simulink model "PIDcontrol_sim"  (R2017a)
settings: Solver=FixedStepAuto  StartTime=0.0  StopTime=Endtime  FixedStep=0.1  RelTol=1e-3
values from neighbouring files (symbols this model uses):
  T_f = 1/omega_c    (= 0.318309886184)    [PIDcontrol.m]
  Ts = 1    [PIDcontrol.m]
undefined symbols (not defined in the file or in its folder): Humusoft, MF644
libraries: sldrtlib x5
settings Model: Creator=CSE2017  LastModifiedBy=CSE2017

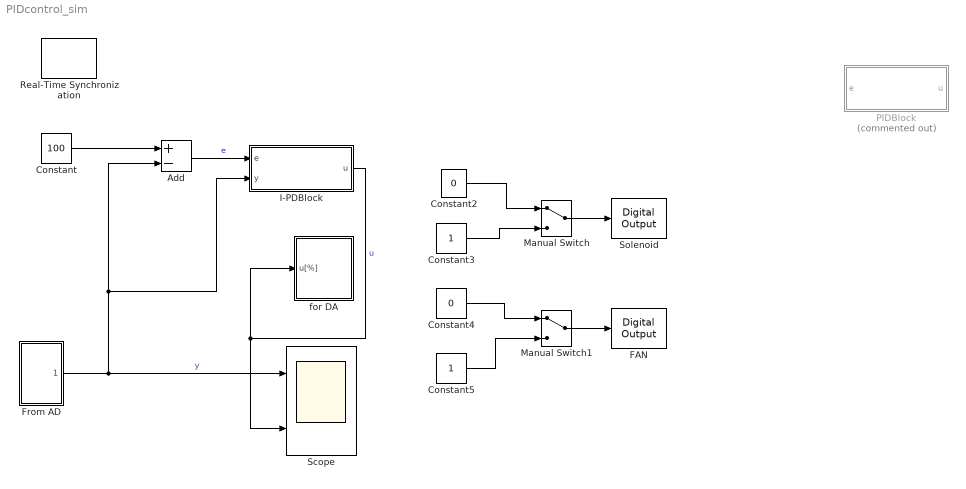
== system PIDcontrol_sim ==
  Add : Sum  Inputs=+-
  Constant : Constant  Value=100
  Constant2 : Constant  Value=0
  Constant3 : Constant
  Constant4 : Constant  Value=0
  Constant5 : Constant
  FAN : sldrtlib/Digital Output  SampleTime=Ts  MaxMissedTicks=10  ShowMissedTicks=off  YieldWhenWaiting=off  DrvName=Humusoft/MF644  DrvAddress=4294967295  DrvOptions=0  Channels=2  BitMode=1  InitialValue=0  FinalValue=1
      settings: AttributesFormatString=Humusoft\nMF644 [auto]  SourceProductName=Simulink Desktop Real-Time  SourceProductBaseCode=WT
  From AD : Subsystem
  I-PDBlock : Subsystem
  Manual Switch : ManualSwitch
  Manual Switch1 : ManualSwitch
  PIDBlock : Subsystem  Commented=on
  Real-Time Synchronization : sldrtlib/Real-Time Synchronization  SampleTime=Ts  MaxMissedTicks=10  ShowMissedTicks=off  YieldWhenWaiting=off
  Scope : Scope  NumInputPorts=2
  Solenoid : sldrtlib/Digital Output  SampleTime=Ts  MaxMissedTicks=10  ShowMissedTicks=off  YieldWhenWaiting=off  DrvName=Humusoft/MF644  DrvAddress=4294967295  DrvOptions=0  Channels=1  BitMode=1  InitialValue=0  FinalValue=0
      settings: AttributesFormatString=Humusoft\nMF644 [auto]  SourceProductName=Simulink Desktop Real-Time  SourceProductBaseCode=WT
  for DA : Subsystem
  wires:
  I-PDBlock/1(u) -> for DA/1(u[%]), Scope/2  "u"
  Constant2/1 -> Manual Switch/1
  Constant3/1 -> Manual Switch/2
  Constant4/1 -> Manual Switch1/1
  Constant5/1 -> Manual Switch1/2
  Manual Switch1/1 -> FAN/1
  Manual Switch/1 -> Solenoid/1
  From AD/1(y[deg.]) -> Add/2, I-PDBlock/2("y "), Scope/1  "y"
  Constant/1 -> Add/1
  Add/1 -> I-PDBlock/1(e)  "e"

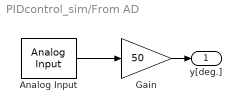
== system PIDcontrol_sim/From AD ==
  Analog Input : sldrtlib/Analog Input  SampleTime=Ts  MaxMissedTicks=10  ShowMissedTicks=off  YieldWhenWaiting=off  DrvName=Humusoft/MF644  DrvAddress=4294967295  DrvOptions=0  Channels=1  RangeMode=1  VoltRange=1  DataType=1
      settings: AttributesFormatString=Humusoft\nMF644 [auto]  SourceProductName=Simulink Desktop Real-Time
  Gain : Gain  Gain=50
  y[deg.] : Outport
  wires:
  Gain/1 -> y[deg.]/1
  Analog Input/1 -> Gain/1

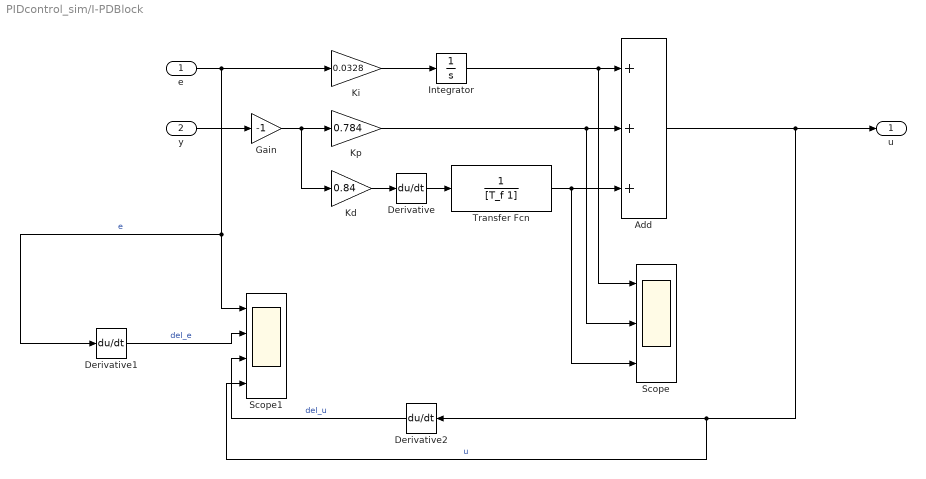
== system PIDcontrol_sim/I-PDBlock ==
  e : Inport
  "y " : Inport  Port=2
  Add : Sum  Inputs=+++
  Derivative : Derivative
  Derivative1 : Derivative
  Derivative2 : Derivative
  Gain : Gain  Gain=-1
  Integrator : Integrator
  Kd : Gain  Gain=0.84
  Ki : Gain  Gain=0.0328
  "Kp " : Gain  Gain=0.784
  Scope : Scope  NumInputPorts=3
  Scope1 : Scope  NumInputPorts=4
  Transfer Fcn : TransferFcn  Denominator=[T_f 1]
  u : Outport
  wires:
  Kd/1 -> Derivative/1
  Ki/1 -> Integrator/1
  "Kp "/1 -> Scope/2, Add/2
  Derivative/1 -> Transfer Fcn/1
  "y "/1 -> Gain/1
  Gain/1 -> Kd/1, "Kp "/1
  Integrator/1 -> Scope/1, Add/1
  Transfer Fcn/1 -> Scope/3, Add/3
  e/1 -> Derivative1/1, Scope1/1, Ki/1  "e"
  Derivative1/1 -> Scope1/2  "del_e"
  Add/1 -> Scope1/4, Derivative2/1, u/1  "u"
  Derivative2/1 -> Scope1/3  "del_u"

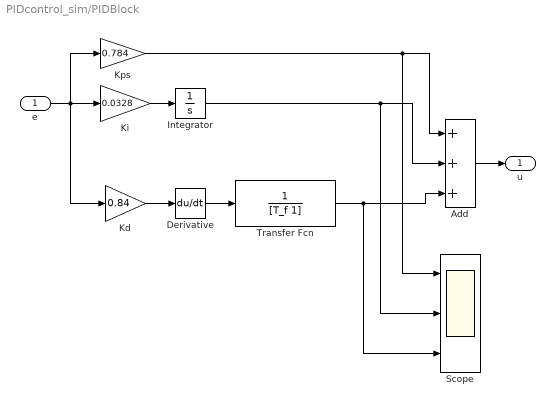
== system PIDcontrol_sim/PIDBlock ==
  e : Inport
  Add : Sum  Inputs=+++
  Derivative : Derivative
  Integrator : Integrator
  Kd : Gain  Gain=0.84
  Ki : Gain  Gain=0.0328
  Kps : Gain  Gain=0.784
  Scope : Scope  NumInputPorts=3
  Transfer Fcn : TransferFcn  Denominator=[T_f 1]
  u : Outport
  wires:
  Ki/1 -> Integrator/1
  Kd/1 -> Derivative/1
  e/1 -> Kps/1, Kd/1, Ki/1
  Integrator/1 -> Scope/2, Add/2
  Derivative/1 -> Transfer Fcn/1
  Add/1 -> u/1
  Kps/1 -> Scope/1, Add/1
  Transfer Fcn/1 -> Scope/3, Add/3

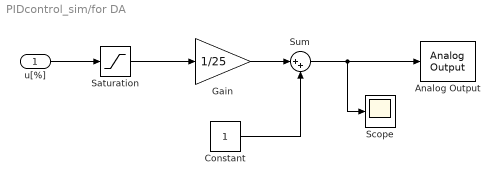
== system PIDcontrol_sim/for DA ==
  u[%] : Inport
  "Analog Output " : sldrtlib/Analog Output  SampleTime=Ts  MaxMissedTicks=10  ShowMissedTicks=off  YieldWhenWaiting=off  DrvName=Humusoft/MF644  DrvAddress=4294967295  DrvOptions=0  Channels=1  RangeMode=1  VoltRange=1  InitialValue=1  FinalValue=1
      settings: AttributesFormatString=Humusoft\nMF644 [auto]  SourceProductName=Simulink Desktop Real-Time
  Constant : Constant
  Gain : Gain  Gain=1/25
  Saturation : Saturate  UpperLimit=100  LowerLimit=0
  Scope : Scope
  Sum : Sum  Inputs=|++
  wires:
  Gain/1 -> Sum/1
  u[%]/1 -> Saturation/1
  Sum/1 -> Scope/1, "Analog Output "/1
  Constant/1 -> Sum/2
  Saturation/1 -> Gain/1
